simulink model "ardupilotsailboat"  (R2022b)
settings: Solver=VariableStepAuto  StartTime=0.0  StopTime=85  RelTol=1e-3
values from neighbouring files (symbols this model uses):
  m11 = 0.1    [ThreeDOF.m]
  m22 = 0.1    [ThreeDOF.m]
undefined symbols (not defined in the file or in its folder): Ixx, m, Waypoints, Yv
libraries: cstblocks x2, simulink x1
(part 1 of 2)
settings Model: Creator=ruben  LastModifiedBy=ruben
settings SolverCC: MaxConsecutiveZCs=10  MaxConsecutiveMinStep=10  ZeroCrossControl=DisableAll  ZeroCrossAlgorithm=Adaptive  SolverResetMethod=Robust
settings DebuggingCC: SignalInfNanChecking=warning  AlgebraicLoopMsg=error  ArtificialAlgebraicLoopMsg=error  BlockPriorityViolationMsg=error  MinStepSizeMsg=error  MaskedZcDiagnostic=error  IgnoredZcDiagnostic=none  MultiTaskCondExecSysMsg=warning  MultiTaskRateTransMsg=warning  CheckMatrixSingularityMsg=error  StateNameClashWarn=warning

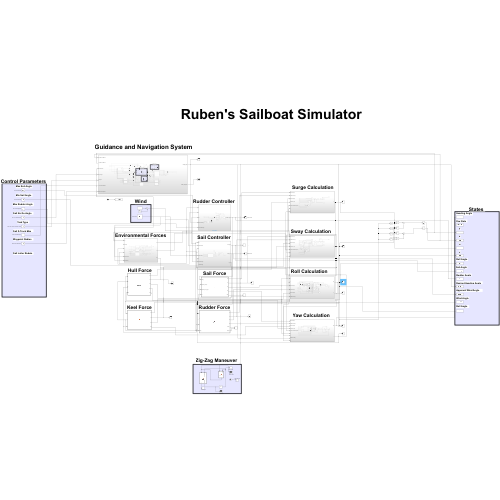
[thumbnail: Simulink's stored preview of the top-level diagram]
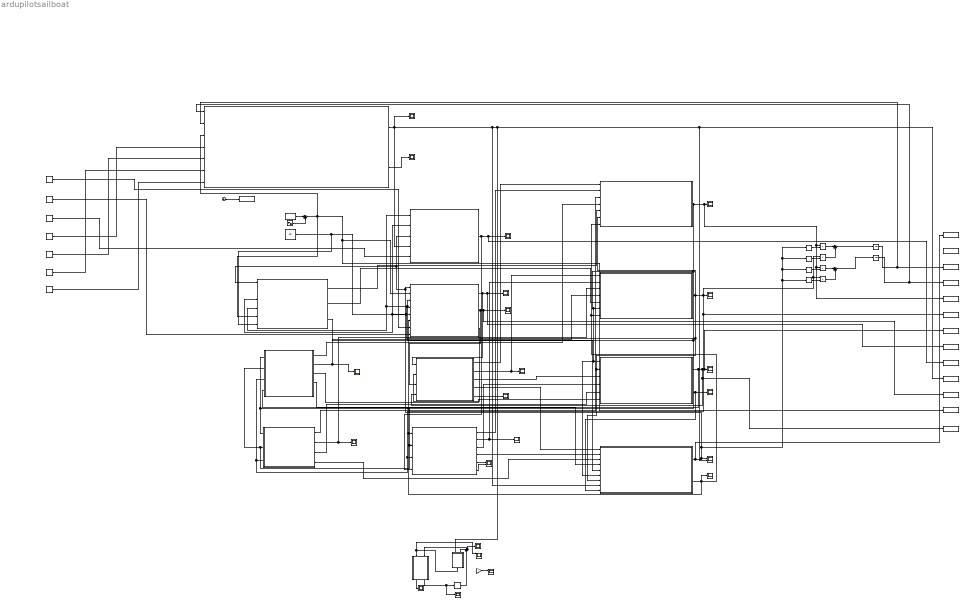
== system ardupilotsailboat ==
  note: Sail Force
  note: Ruben's Sailboat Simulator
  note: States
  note: x
  note: y
  note: Yaw Rate
  note: Heading Angle
  note: u
  note: v
  note: Roll Angle
  note: Sail Angle
  note: Rudder Angle
  note: Desired Heading Angle
  note: Apparent Wind Angle
  note: Wind Angle
  note: Roll Angle
  note: Guidance and Navigation System
  note: Environmental Forces
  note: Surge Calculation
  note: Sway Calculation
  note: Roll Calculation
  note: Yaw Calculation
  note: Wind
  note: Rudder Force
  note: Keel Force
  note: Hull Force
  note: Sail Controller
  note: Rudder Controller
  note: Zig-Zag Maneuver
  note: Control Parameters
  note: Max Sail Angle
  note: Min Sail Angle
  note: Sail No Go Angle
  note: Sail X-Track Max
  note: Sail Loiter Raduis
  note: Waypoint Radius
  note: Tack Type
  note: Max Rudder Angle
  Clock2 : Clock
  Cross-Track Distance(m) : Constant  Value=10
  Delay1 : Delay  DelayLength=1  SampleTime=0.01
  Gain2 : Gain  Gain=180/pi
  Integrator1 : Integrator
  Integrator2 : Integrator
  MATLAB Function3 : MATLAB Function  TreatAsAtomicUnit=on
  MATLAB Function4 : MATLAB Function  TreatAsAtomicUnit=on
  MATLAB Function5 : MATLAB Function  TreatAsAtomicUnit=on
  MATLAB Function6 : MATLAB Function  TreatAsAtomicUnit=on
  MATLAB Function7 : MATLAB Function  TreatAsAtomicUnit=on
  MATLAB Function8 : MATLAB Function  TreatAsAtomicUnit=on
  Product{,1,8..9} (4 alike) : Product
  Radius of Acceptance(m) : Constant  Value=5
  Scope{,1..4,33,35..38,40,42} (12 alike) : Scope
  Scope39 : Scope  NumInputPorts=2
  Scope41 : Scope  NumInputPorts=2
  Sine Wave : Sin  Amplitude=0  Frequency=0.1  SampleTime=0
  Subsystem1 : Subsystem
  Subsystem2 : Subsystem
  Subsystem3 : Subsystem
  Subsystem4 : Subsystem
  Subsystem5 : Subsystem
  Subsystem6 : Subsystem
  Subsystem7 : Subsystem
  Subsystem8 : Subsystem
  Sum : Sum  Inputs=|++
  Sum6 : Sum  Inputs=|+-
  Sum7 : Sum  Inputs=|++
  "Tack Type (1:Direct, 2:Indirect 3:Zone)" : Constant  Value=2
  To Workspace : ToWorkspace  VariableName=yawrate  SaveFormat=Timeseries  SampleTime=-1
  To Workspace1 : ToWorkspace  VariableName=yaw  SaveFormat=Timeseries  SampleTime=-1
  To Workspace10 : ToWorkspace  VariableName=psid  SaveFormat=Timeseries  SampleTime=-1
  To Workspace11 : ToWorkspace  VariableName=awa  SaveFormat=Timeseries  SampleTime=-1
  To Workspace12 : ToWorkspace  VariableName=wind  SaveFormat=Timeseries  SampleTime=-1
  To Workspace13 : ToWorkspace  VariableName=roll  SaveFormat=Timeseries  SampleTime=-1
  To Workspace14 : ToWorkspace  VariableName=time1  SaveFormat=Timeseries  SampleTime=-1
  To Workspace3 : ToWorkspace  VariableName=x  SaveFormat=Timeseries  SampleTime=-1
  To Workspace4 : ToWorkspace  VariableName=y  SaveFormat=Timeseries  SampleTime=-1
  To Workspace5 : ToWorkspace  VariableName=u  SaveFormat=Timeseries  SampleTime=-1
  To Workspace6 : ToWorkspace  VariableName=v  SaveFormat=Timeseries  SampleTime=-1
  To Workspace7 : ToWorkspace  VariableName=phi  SaveFormat=Timeseries  SampleTime=-1
  To Workspace8 : ToWorkspace  VariableName=delta_s  SaveFormat=Timeseries  SampleTime=-1
  To Workspace9 : ToWorkspace  VariableName=delta_r  SaveFormat=Timeseries  SampleTime=-1
  Trigonometric Function : Trigonometry
  Trigonometric Function1 : Trigonometry  Operator=cos
  Trigonometric Function6 : Trigonometry  Operator=cos
  Trigonometric Function7 : Trigonometry
  apparent wind : Scope
  max rudder angle(Rad) : Constant  Value=pi/6
  max sail angle(Rad) : Constant  Value=pi/3
  min sail angle(Rad) : Constant  Value=-pi/3
  rudder and psi1 : Scope  NumInputPorts=2
  rudder angle5 : Scope
  rudder angle6 : Scope
  rudder angle7 : Scope  NumInputPorts=3
  rudder angle8 : Scope
  rudder_angle1 : Scope
  sail angle : Scope
  sail no go angle(Degrees) : Constant  Value=45
  wind direction : Constant  Value=pi/2-0.01
  wind velocity : Constant  Value=10
  wires:
  Trigonometric Function1/1 -> Product/2
  Trigonometric Function/1 -> Product1/2
  Product/1 -> Sum6/1
  Product1/1 -> Sum6/2
  Sum6/1 -> Integrator1/1
  Product9/1 -> Sum7/2
  Product8/1 -> Sum7/1
  Trigonometric Function7/1 -> Product8/2
  Trigonometric Function6/1 -> Product9/2
  Sum7/1 -> Integrator2/1
  Integrator2/1 -> Subsystem1/1(x position of Sailboat), To Workspace3/1
  Integrator1/1 -> Subsystem1/2(y position of Sailboat), To Workspace4/1
  Subsystem1/1(heading (rad)) -> To Workspace10/1, Scope39/2, MATLAB Function8/1(psi), Subsystem6/8(desired heading), Scope/1, Subsystem8/4(desired heading)
  Subsystem1/2(heading (degrees)) -> Scope33/1
  MATLAB Function3/1(Xs) -> Subsystem2/1(sail force (Xs))
  MATLAB Function3/2(Ys) -> Scope1/1, Subsystem4/1(sail force (Ys))
  MATLAB Function3/3(Ks) -> Subsystem5/3(sail force (Ks))
  MATLAB Function3/4(Ns) -> Subsystem6/1(sail force (Ns))
  MATLAB Function4/1(Xr) -> Subsystem2/2(rudder force (Xr))
  MATLAB Function4/2(Yr) -> Scope2/1, Subsystem4/2(rudder force (Yr))
  MATLAB Function4/3(Kr) -> Subsystem5/4(hull force(Kh))
  MATLAB Function4/4(Nr) -> Subsystem6/2(rudder force (Nr))
  MATLAB Function5/1(Xk) -> Subsystem2/3(keel force (Xk))
  MATLAB Function5/2(Yk) -> Scope3/1, Subsystem4/3(keel force (Yk))
  MATLAB Function5/3(Kk) -> Subsystem5/5(keel force (Kk))
  MATLAB Function5/4(Nk) -> Subsystem6/3(keel force (Nk))
  MATLAB Function6/1(Xh) -> Subsystem2/4(hull force (Xh))
  MATLAB Function6/3(Kh) -> Subsystem5/6(rudder force (Kr))
  MATLAB Function6/4(Nh) -> Subsystem6/4(hull force (Nh))
  Subsystem4/1(v) -> To Workspace6/1, MATLAB Function6/3(v), MATLAB Function5/3(v), MATLAB Function4/3(v), Product1/1, Product9/1, Scope36/1, Subsystem2/6(v), Subsystem6/7(v), Subsystem5/2(v), Subsystem8/2(v), Subsystem3/3(v), Subsystem7/4(v)
  Subsystem3/1(Xe) -> Subsystem2/5(environmental force (Xe))
  Subsystem3/2(Ye) -> Subsystem4/5(environmental force (Ye))
  Subsystem3/3(Ne) -> Subsystem6/5(environmental force (Ne))
  Subsystem2/1(u) -> MATLAB Function5/2(u), MATLAB Function6/2(u), MATLAB Function4/2(u), Subsystem8/1(u), Subsystem3/4(u), Subsystem7/3(u), Subsystem6/6(u), Subsystem5/1(u), Subsystem4/6(u), To Workspace5/1, Product8/1, Product/1, Scope35/1
  Subsystem6/2(r) -> Subsystem7/6(r), MATLAB Function5/1(r), MATLAB Function6/1(r), MATLAB Function4/1(r), Scope40/1, Subsystem2/7(r), Subsystem4/7(r)
  Subsystem5/2(p) -> Subsystem6/9(p), Scope38/1
  Subsystem5/1(phi) -> MATLAB Function6/4(phi), To Workspace13/1, MATLAB Function3/4(phi), To Workspace7/1, Scope37/1
  Clock2/1 -> To Workspace14/1
  MATLAB Function7/2(nextState) -> rudder angle5/1, Delay1/1
  Delay1/1 -> rudder angle8/1, MATLAB Function8/2(state), MATLAB Function7/2(currentState)
  MATLAB Function7/1(y) -> rudder angle6/1
  MATLAB Function8/1(y) -> MATLAB Function7/1(r), rudder angle7/1
  Gain2/1 -> rudder and psi1/1
  Sum/1 -> Subsystem3/5(wind Direction), Subsystem1/3(wind Direction), To Workspace12/1, Subsystem7/2(wind direction)
  wind velocity/1 -> Subsystem3/6(wind Velocity), Subsystem7/5(wind velocity)
  Subsystem7/1(sail angle) -> MATLAB Function3/1(delta_s), To Workspace8/1, sail angle/1
  Subsystem7/2(alpha_aw) -> To Workspace11/1, apparent wind/1, MATLAB Function3/3(apparent_wind_angle)
  Subsystem7/3(V_aw) -> MATLAB Function3/2(apparent_velocity)
  Subsystem8/1(rudder angle) -> To Workspace9/1, rudder_angle1/1, MATLAB Function4/4("delta_r ")
  MATLAB Function4/5(delta_r) -> Scope41/1
  MATLAB Function4/6(alpha_a) -> Scope41/2
  MATLAB Function3/5(awa) -> Scope42/1
  Subsystem6/1(psi) -> To Workspace1/1, Trigonometric Function7/1, Trigonometric Function/1, Trigonometric Function1/1, Trigonometric Function6/1, Subsystem7/1(psi), Subsystem3/1(psi), Subsystem8/3(psi), Scope39/1
  MATLAB Function6/2(Yh) -> Subsystem4/4(hull force (Yh)), Scope4/1
  max sail angle(Rad)/1 -> Subsystem7/7(max sail angle)
  min sail angle(Rad)/1 -> Subsystem7/8(min sail angle)
  max rudder angle(Rad)/1 -> Subsystem8/5(max rudder angle)
  sail no go angle(Degrees)/1 -> Subsystem1/4(no go Angle)
  "Tack Type (1:Direct, 2:Indirect 3:Zone)"/1 -> Subsystem1/5(tack Type)
  Cross-Track Distance(m)/1 -> Subsystem1/6(Cross-Track Distance)
  Radius of Acceptance(m)/1 -> Subsystem1/7(radius of acceptance)
  wind direction/1 -> Sum/1
  Sine Wave/1 -> Sum/2

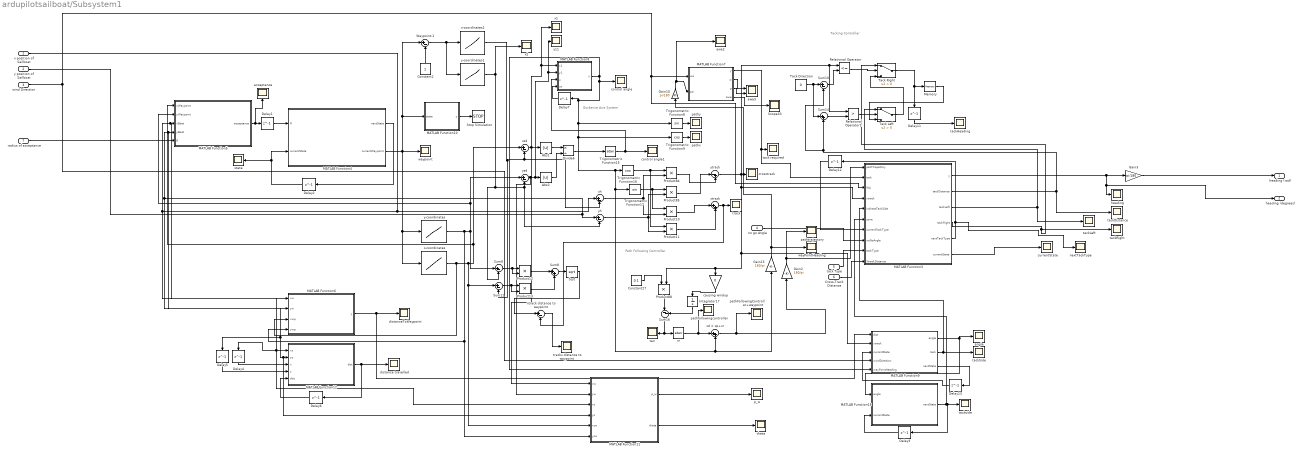
== system ardupilotsailboat/Subsystem1 ==
  note: Guidance Axis System
  note: Tacking Controller
  note: Path Following Controller
  x position of Sailboat : Inport
  y position of Sailboat : Inport  Port=2
  wind Direction : Inport  Port=3
  no go Angle : Inport  Port=4
  tack Type : Inport  Port=5
  Cross-Track Distance : Inport  Port=6
  radius of acceptance : Inport  Port=7
  Abs1 : Abs  SaturateOnIntegerOverflow=off
  Abs2 : Abs  SaturateOnIntegerOverflow=off
  Constant2 : Constant
  Constant27 : Constant  Value=0.1
  Delay{1..2,4..7,11..12} (8 alike) : Delay  DelayLength=1
  Delay13 : Delay  DelayLength=1  SampleTime=2
  Delay3 : Delay  DelayLength=1  SampleTime=2
  Divide6 : Product  Inputs=*/
  Gain10 : Gain  Gain=pi/180
  Gain15 : Gain  Gain=180/pi
  Gain2 : Gain  Gain=180/pi
  Gain3 : Gain  Gain=pi/180
  Integrator17 : Integrator  LimitOutput=on  UpperSaturationLimit=10  LowerSaturationLimit=-10
  MATLAB Function10 : MATLAB Function  TreatAsAtomicUnit=on
  MATLAB Function11 : MATLAB Function  TreatAsAtomicUnit=on
  MATLAB Function12 : MATLAB Function  TreatAsAtomicUnit=on
  MATLAB Function18 : MATLAB Function  TreatAsAtomicUnit=on
  MATLAB Function3 : MATLAB Function  TreatAsAtomicUnit=on
  MATLAB Function4 : MATLAB Function  TreatAsAtomicUnit=on
  MATLAB Function5 : MATLAB Function  TreatAsAtomicUnit=on
  MATLAB Function6 : MATLAB Function  TreatAsAtomicUnit=on
  MATLAB Function7 : MATLAB Function  TreatAsAtomicUnit=on
  MATLAB Function8 : MATLAB Function  TreatAsAtomicUnit=on
  MATLAB Function9 : MATLAB Function  TreatAsAtomicUnit=on
  Memory : Memory
  Product{10..13,84..85,88} (7 alike) : Product
  Relational Operator : RelationalOperator  Operator=<=  OutDataTypeStr=boolean  RndMeth=Simplest  InputSameDT=off
  Relational Operator1 : RelationalOperator  Operator=>  OutDataTypeStr=boolean  RndMeth=Simplest  InputSameDT=off
  Scope33 : Scope
  Sqrt : Sqrt
  Stop Simulation : Stop
  Sum10 : Sum  Inputs=|+-
  Sum11 : Sum  Inputs=|+-
  Sum14 : Sum  Inputs=|++
  Sum16 : Sum  Inputs=|--
  Sum8 : Sum  Inputs=|++
  Sum9 : Sum  Inputs=|+-
  Tack Direction : Constant  Value=0
  Tack Left : Switch  Criteria=u2 > Threshold  SaturateOnIntegerOverflow=off  InputSameDT=off
  Tack Right : Switch  Criteria=u2 > Threshold  SaturateOnIntegerOverflow=off  InputSameDT=off
  Trigonometric Function15 : Trigonometry  Operator=atan
  Trigonometric Function16 : Trigonometry  Operator=cos
  Trigonometric Function17 : Trigonometry
  Trigonometric Function8 : Trigonometry
  Trigonometric Function9 : Trigonometry  Operator=cos
  Waypoint-1 : Sum  Inputs=|+-
  acceptance : Scope
  angle : Scope
  awa2 : Scope
  awa3 : Scope  NumInputPorts=2
  causing windup : Gain  Gain=0
  control angle : Scope
  control angle1 : Scope
  crosstrack : Scope
  currentState : Scope
  distance travelled : Scope
  distanceToWaypoint : Scope
  heading : Scope
  nextTackType : Scope
  p_w : Scope
  "pathFollowingController+waypoint " : Scope
  pathfollowingcontroller : Scope
  pathtrajectory : Scope
  pathx : Scope
  pathy : Scope
  state : Scope
  tack required : Scope
  tackDistance : Scope
  tackHeading : Scope
  tackLeft : Scope
  tackRight : Scope
  tackSide : Scope
  tackside : Scope
  tan : Scope
  theta : Scope
  track : Scope
  trackx distance to waypoint : Scope
  wayPointHeading : Scope
  waypoint : Scope
  x-coordinates : Lookup_n-D  NumberOfTableDimensions=1  BreakpointsForDimension1=Waypoints.number  Table=Waypoints.x  InterpMethod=Cubic spline  ExtrapMethod=Cubic spline  InternalRulePriority=Speed  RndMeth=Simplest
  x-coordinates1 : Lookup_n-D  NumberOfTableDimensions=1  BreakpointsForDimension1=Waypoints.number  Table=Waypoints.x  InterpMethod=Cubic spline  ExtrapMethod=Cubic spline  InternalRulePriority=Speed  RndMeth=Simplest
  x1 : Scope
  x2 : Scope
  xd = xp+xr : Sum  Inputs=|++
  xh : Sum  Inputs=|+-
  xr : Trigonometry  Operator=atan
  xsd : Sum  Inputs=|+-
  xtrack : Sum  Inputs=|++
  xtrack distance to waypoint : Sum  Inputs=|+-
  y-coordinates : Lookup_n-D  NumberOfTableDimensions=1  BreakpointsForDimension1=Waypoints.number  Table=Waypoints.y  InterpMethod=Cubic spline  ExtrapMethod=Cubic spline  InternalRulePriority=Speed  RndMeth=Simplest
  y-coordinates1 : Lookup_n-D  NumberOfTableDimensions=1  BreakpointsForDimension1=Waypoints.number  Table=Waypoints.y  InterpMethod=Cubic spline  ExtrapMethod=Cubic spline  InternalRulePriority=Speed  RndMeth=Simplest
  y11 : Scope
  yh : Sum  Inputs=|+-
  ysd : Sum  Inputs=|+-
  ytrack : Sum  Inputs=|-+
  heading (rad) : Outport
  heading (degrees) : Outport  Port=2
  wires:
  MATLAB Function11/2(theta) -> theta/1
  MATLAB Function7/3(p) -> awa3/2
  Delay2/1 -> MATLAB Function4/2(currentState), state/1
  y-coordinates/1 -> MATLAB Function11/6(ycw), MATLAB Function6/4(ywp), MATLAB Function5/2(yWaypoint), ysd/1, Sum9/1
  Trigonometric Function17/1 -> Product10/1, Product85/1
  MATLAB Function3/6(currentState) -> currentState/1
  MATLAB Function3/1(y) -> heading (degrees)/1, heading/1, Gain3/1
  Gain2/1 -> MATLAB Function3/1(pathTrajectory), pathtrajectory/1
  Delay12/1 -> MATLAB Function3/7(currentTackType)
  MATLAB Function4/2(currentWaypoint) -> MATLAB Function10/1(state), Waypoint-1/1, waypoint/1, x-coordinates/1, y-coordinates/1
  yh/1 -> Product85/2, Product11/2
  MATLAB Function7/2(w) -> awa3/1
  Sum14/1 -> Relational Operator1/2
  y position of Sailboat/1 -> yh/1, MATLAB Function6/2(yw), MATLAB Function5/4(yBoat), MATLAB Function11/4(ys), MATLAB Function12/2(ys), Delay5/1
  ytrack/1 -> MATLAB Function3/4(xtrack), Product88/2, causing windup/1, MATLAB Function9/2(xtrack), crosstrack/1, Relational Operator1/1, Relational Operator/1
  Product85/1 -> ytrack/1
  Delay11/1 -> tackHeading/1
  MATLAB Function3/2(tackDistance) -> Sum10/2, Sum14/2, tackDistance/1
  Integrator17/1 -> Sum16/2
  Abs1/1 -> Divide6/1
  Trigonometric Function16/1 -> Product11/1, Product84/1
  Delay7/1 -> MATLAB Function8/4(us)
  MATLAB Function18/1(nextState) -> tackside/1, Delay3/1, MATLAB Function3/6(zone)
  xd = xp+xr/1 -> "pathFollowingController+waypoint "/1, Gain2/1
  Gain10/1 -> MATLAB Function7/2(psi), awa2/1
  MATLAB Function3/5(nextTackType) -> nextTackType/1, Delay12/1
  Delay13/1 -> MATLAB Function9/3(currentState)
  Waypoint-1/1 -> x-coordinates1/1, y-coordinates1/1
  Delay3/1 -> MATLAB Function18/2(currentState)
  xsd/1 -> MATLAB Function11/1(xw), MATLAB Function8/1(x1), x1/1, Abs1/1
  Constant2/1 -> Waypoint-1/2
  MATLAB Function8/1(y) -> Trigonometric Function8/1, Trigonometric Function9/1, Trigonometric Function17/1, xd = xp+xr/2, Gain15/1, Trigonometric Function16/1, Delay7/1, control angle/1, MATLAB Function9/5(wayPointHeading)
  xh/1 -> Product84/2, Product10/2
  Delay1/1 -> MATLAB Function4/1(R)
  MATLAB Function9/3(nextState) -> Delay13/1
  Product84/1 -> ytrack/2
  y-coordinates1/1 -> yh/2, ysd/2, Sum9/2, x2/1
  x position of Sailboat/1 -> xh/1, MATLAB Function11/3(xs), MATLAB Function12/1(xs), Delay4/1, MATLAB Function6/1(xw), MATLAB Function5/3(xBoat)
  Trigonometric Function15/1 -> control angle1/1, MATLAB Function8/3(u)
  ysd/1 -> y11/1, MATLAB Function8/2(y1), Abs2/1, MATLAB Function11/2(yw)
  x-coordinates1/1 -> Sum11/2, xh/2, xsd/2
  Sum16/1 -> xr/1, tan/1
  Divide6/1 -> Trigonometric Function15/1
  Product13/1 -> Sum8/2
  Gain15/1 -> Gain10/1, wayPointHeading/1
  MATLAB Function6/1(y) -> MATLAB Function9/1(dist), distanceToWaypoint/1
  Delay5/1 -> MATLAB Function12/4(y)
  MATLAB Function9/1(angle) -> angle/1, MATLAB Function18/1(angle)
  Product88/1 -> Sum16/1
  Relational Operator1/1 -> Tack Left/2
  MATLAB Function3/3(tackLeft) -> Tack Left/1, tackLeft/1
  Tack Right/1 -> Memory/1, Delay11/1
  xtrack distance to waypoint/1 -> trackx distance to waypoint/1
  x-coordinates/1 -> MATLAB Function6/3(xwp), MATLAB Function11/5(xcw), Sum11/1, xsd/1, MATLAB Function5/1(xWaypoint)
  Constant27/1 -> Product88/1
  Memory/1 -> Tack Left/3
  Product11/1 -> xtrack/2
  Trigonometric Function8/1 -> pathy/1
  MATLAB Function7/1(y) -> MATLAB Function3/2(tack), tack required/1
  Delay4/1 -> MATLAB Function12/3(x)
  causing windup/1 -> Integrator17/1
  Tack Left/1 -> Tack Right/3
  MATLAB Function9/2(tack) -> MATLAB Function3/5(indirectTackSide), tackSide/1
  MATLAB Function10/1(y) -> Stop Simulation/1
  wind Direction/1 -> MATLAB Function3/3(WA), MATLAB Function7/1(wa), MATLAB Function9/4(windDirection)
  Sum8/1 -> Sqrt/1
  Sum11/1 -> Product13/2, Product13/1
  Tack Direction/1 -> Sum14/1, Sum10/1
  Sum9/1 -> Product12/1, Product12/2
  Delay6/1 -> MATLAB Function12/5("dist ")
  MATLAB Function5/1(acceptance) -> acceptance/1, Delay1/1
  MATLAB Function12/1(dist) -> distance travelled/1, Delay6/1
  Relational Operator/1 -> Tack Right/2
  Sum10/1 -> Relational Operator/2
  xtrack/1 -> xtrack distance to waypoint/2, track/1
  Abs2/1 -> Divide6/2
  MATLAB Function4/1(nextState) -> Delay2/1
  Sqrt/1 -> xtrack distance to waypoint/1
  MATLAB Function11/1(p_w) -> p_w/1
  Product10/1 -> xtrack/1
  xr/1 -> xd = xp+xr/1, pathfollowingcontroller/1
  MATLAB Function3/4(tackRight) -> Tack Right/1, tackRight/1
  Product12/1 -> Sum8/1
  Trigonometric Function9/1 -> pathx/1
  Gain3/1 -> heading (rad)/1
  MATLAB Function7/4(awa) -> Scope33/1
  no go Angle/1 -> MATLAB Function3/8(noGoAngle)
  tack Type/1 -> MATLAB Function3/9(tackType)
  Cross-Track Distance/1 -> MATLAB Function3/10(XtrackDistance)
  radius of acceptance/1 -> MATLAB Function5/5(R)

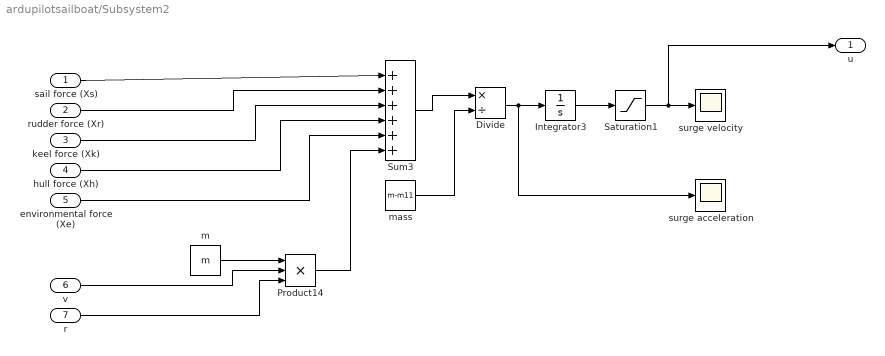
== system ardupilotsailboat/Subsystem2 ==
  sail force (Xs) : Inport
  rudder force (Xr) : Inport  Port=2
  keel force (Xk) : Inport  Port=3
  hull force (Xh) : Inport  Port=4
  environmental force (Xe) : Inport  Port=5
  v : Inport  Port=6
  r : Inport  Port=7
  Divide : Product  Inputs=*/
  Integrator3 : Integrator  InitialCondition=1.3
  Product14 : Product  Inputs=3
  Saturation1 : Saturate  UpperLimit=1.3  LowerLimit=-1.3
  Sum3 : Sum  Inputs=|++++++
  m : Constant  Value=m
  mass : Constant  Value=m-m11
  surge acceleration : Scope
  surge velocity : Scope
  u : Outport
  wires:
  Saturation1/1 -> u/1, surge velocity/1
  sail force (Xs)/1 -> Sum3/1
  Integrator3/1 -> Saturation1/1
  m/1 -> Product14/1
  Divide/1 -> surge acceleration/1, Integrator3/1
  mass/1 -> Divide/2
  Sum3/1 -> Divide/1
  Product14/1 -> Sum3/6
  rudder force (Xr)/1 -> Sum3/2
  keel force (Xk)/1 -> Sum3/3
  hull force (Xh)/1 -> Sum3/4
  environmental force (Xe)/1 -> Sum3/5
  v/1 -> Product14/2
  r/1 -> Product14/3

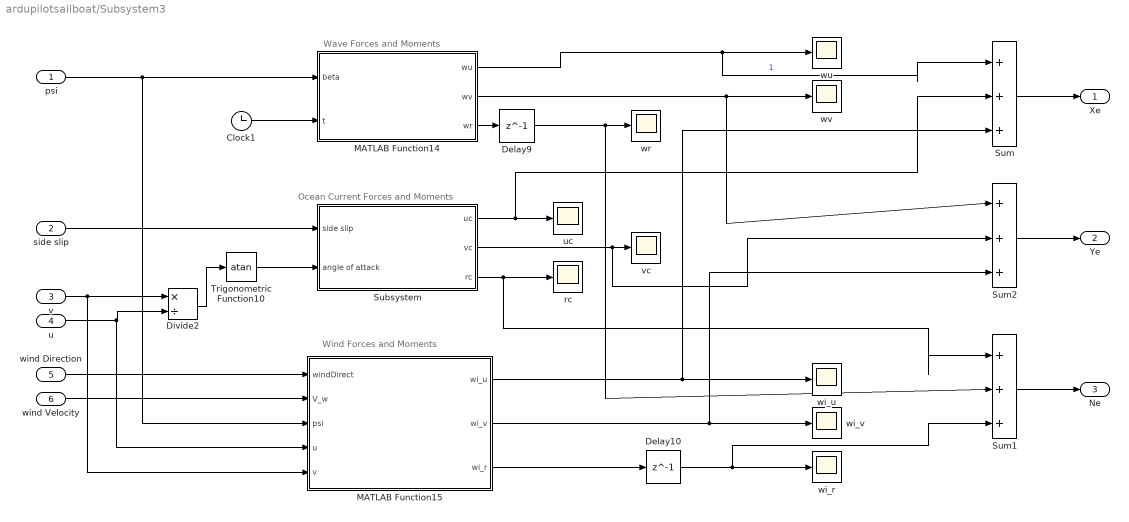
== system ardupilotsailboat/Subsystem3 ==
  note: Wave Forces and Moments
  note: Wind Forces and Moments
  note: Ocean Current Forces and Moments
  psi : Inport
  side slip : Inport  Port=2
  v : Inport  Port=3
  u : Inport  Port=4
  wind Direction : Inport  Port=5
  wind Velocity : Inport  Port=6
  Clock1 : Clock
  Delay10 : Delay  DelayLength=1
  Delay9 : Delay  DelayLength=1
  Divide2 : Product  Inputs=*/
  MATLAB Function14 : MATLAB Function  TreatAsAtomicUnit=on
  MATLAB Function15 : MATLAB Function  TreatAsAtomicUnit=on
  Subsystem : Subsystem
  Sum : Sum  Inputs=|+++
  Sum1 : Sum  Inputs=|+++
  Sum2 : Sum  Inputs=|+++
  Trigonometric Function10 : Trigonometry  Operator=atan
  rc : Scope
  uc : Scope
  vc : Scope
  wi_r : Scope
  wi_u : Scope
  wi_v : Scope
  wr : Scope
  wu : Scope
  wv : Scope
  Xe : Outport
  Ye : Outport  Port=2
  Ne : Outport  Port=3
  wires:
  MATLAB Function14/2(wv) -> Sum2/1, wv/1
  Trigonometric Function10/1 -> Subsystem/2(angle of attack)
  MATLAB Function14/3(wr) -> Delay9/1
  MATLAB Function15/2(wi_v) -> Sum2/3, wi_v/1
  Subsystem/1(uc) -> Sum/2, uc/1
  MATLAB Function15/3(wi_r) -> Delay10/1
  MATLAB Function15/1(wi_u) -> Sum/3, wi_u/1
  Clock1/1 -> MATLAB Function14/2(t)
  Subsystem/2(vc) -> Sum2/2, vc/1
  MATLAB Function14/1(wu) -> Sum/1, wu/1  "1"
  Divide2/1 -> Trigonometric Function10/1
  psi/1 -> MATLAB Function14/1(beta), MATLAB Function15/3(psi)
  side slip/1 -> Subsystem/1(side slip)
  v/1 -> MATLAB Function15/5(v), Divide2/1
  u/1 -> MATLAB Function15/4(u), Divide2/2
  wind Direction/1 -> MATLAB Function15/1(windDirect)
  wind Velocity/1 -> MATLAB Function15/2(V_w)
  Sum/1 -> Xe/1
  Sum1/1 -> Ne/1
  Sum2/1 -> Ye/1
  Delay10/1 -> Sum1/3, wi_r/1
  Subsystem/3(rc) -> Sum1/1, rc/1
  Delay9/1 -> Sum1/2, wr/1

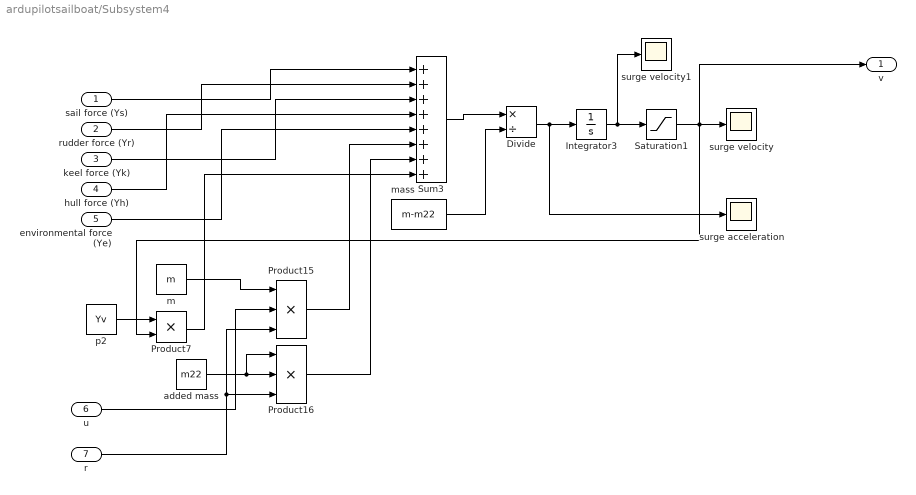
== system ardupilotsailboat/Subsystem4 ==
  sail force (Ys) : Inport
  rudder force (Yr) : Inport  Port=2
  keel force (Yk) : Inport  Port=3
  hull force (Yh) : Inport  Port=4
  environmental force (Ye) : Inport  Port=5
  u : Inport  Port=6
  r : Inport  Port=7
  Divide : Product  Inputs=*/
  Integrator3 : Integrator  LimitOutput=on  UpperSaturationLimit=0.05  LowerSaturationLimit=-0.05
  Product15 : Product  Inputs=3
  Product16 : Product  Inputs=3
  Product7 : Product
  Saturation1 : Saturate  UpperLimit=0.1  LowerLimit=-0.1
  Sum3 : Sum  Inputs=|++++++++
  added mass : Constant  Value=m22
  m : Constant  Value=m
  mass : Constant  Value=m-m22
  p2 : Constant  Value=Yv
  surge acceleration : Scope
  surge velocity : Scope
  surge velocity1 : Scope
  v : Outport
  wires:
  Saturation1/1 -> Product7/2, v/1, surge velocity/1
  sail force (Ys)/1 -> Sum3/1
  Integrator3/1 -> surge velocity1/1, Saturation1/1
  Divide/1 -> surge acceleration/1, Integrator3/1
  mass/1 -> Divide/2
  Sum3/1 -> Divide/1
  rudder force (Yr)/1 -> Sum3/2
  keel force (Yk)/1 -> Sum3/3
  hull force (Yh)/1 -> Sum3/4
  environmental force (Ye)/1 -> Sum3/5
  added mass/1 -> Product16/1, Product16/2
  p2/1 -> Product7/1
  m/1 -> Product15/1
  Product15/1 -> Sum3/6
  Product16/1 -> Sum3/7
  u/1 -> Product15/2
  Product7/1 -> Sum3/8
  r/1 -> Product16/3, Product15/3

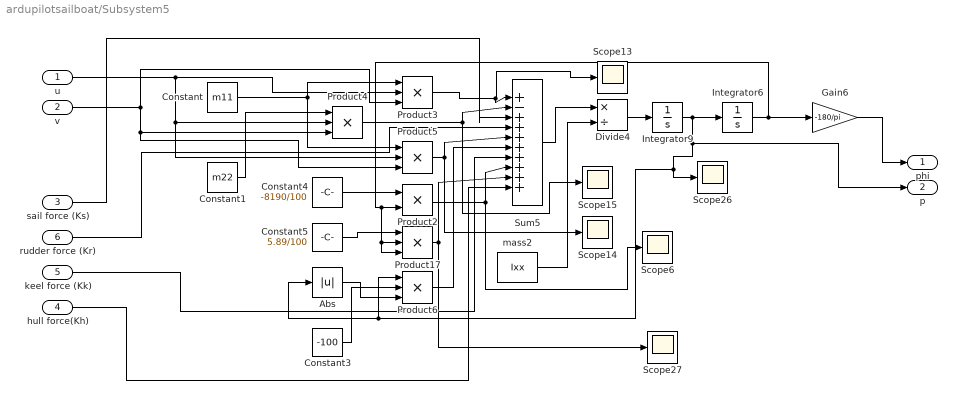
== system ardupilotsailboat/Subsystem5 ==
  u : Inport
  v : Inport  Port=2
  sail force (Ks) : Inport  Port=3
  hull force(Kh) : Inport  Port=4
  keel force (Kk) : Inport  Port=5
  rudder force (Kr) : Inport  Port=6
  Abs : Abs  SaturateOnIntegerOverflow=off
  Constant : Constant  Value=m11
  Constant1 : Constant  Value=m22
  Constant3 : Constant  Value=-100
  Constant4 : Constant  Value=-8190/100
  Constant5 : Constant  Value=5.89/100
  Divide4 : Product  Inputs=*/
  Gain6 : Gain  Gain=-180/pi
  Integrator6 : Integrator
  Integrator9 : Integrator
  Product{3..6,17} (5 alike) : Product  Inputs=3
  Product2 : Product
  Scope{6,13..15,26..27} (6 alike) : Scope
  Sum5 : Sum  Inputs=|+-++++++++
  mass2 : Constant  Value=Ixx
  phi : Outport
  p : Outport  Port=2
  wires:
  Product6/1 -> Sum5/6
  Abs/1 -> Product6/3
  Product4/1 -> Scope15/1, Sum5/2
  Constant3/1 -> Product6/2
  Integrator9/1 -> p/1, Abs/1, Product6/1, Scope26/1, Integrator6/1
  Integrator6/1 -> Product2/2, Product17/3, Product17/2, Gain6/1
  Product17/1 -> Sum5/9, Scope27/1
  Product2/1 -> Scope6/1, Sum5/8
  Constant/1 -> Product5/1, Product3/1
  Product3/1 -> Sum5/1, Scope13/1
  Constant5/1 -> Product17/1
  Product5/1 -> Scope14/1, Sum5/5
  Constant4/1 -> Product2/1
  Divide4/1 -> Integrator9/1
  mass2/1 -> Divide4/2
  Constant1/1 -> Product4/1
  Sum5/1 -> Divide4/1
  u/1 -> Product5/2, Product4/2, Product3/2
  v/1 -> Product3/3, Product5/3, Product4/3
  sail force (Ks)/1 -> Sum5/3
  rudder force (Kr)/1 -> Sum5/4
  keel force (Kk)/1 -> Sum5/7
  hull force(Kh)/1 -> Sum5/10
  Gain6/1 -> phi/1

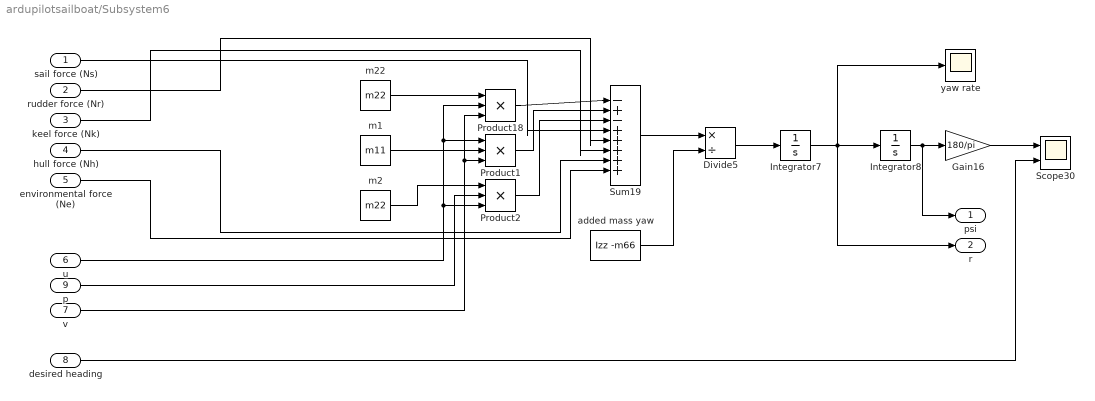
== system ardupilotsailboat/Subsystem6 ==
  sail force (Ns) : Inport
  rudder force (Nr) : Inport  Port=2
  keel force (Nk) : Inport  Port=3
  hull force (Nh) : Inport  Port=4
  environmental force (Ne) : Inport  Port=5
  u : Inport  Port=6
  v : Inport  Port=7
  desired heading : Inport  Port=8
  p : Inport  Port=9
  Divide5 : Product  Inputs=*/
  Gain16 : Gain  Gain=180/pi
  Integrator7 : Integrator
  Integrator8 : Integrator
  Product1 : Product  Inputs=3
  Product18 : Product  Inputs=3
  Product2 : Product  Inputs=3
  Scope30 : Scope  NumInputPorts=2
  Sum19 : Sum  Inputs=|-+-+++++
  added mass yaw : Constant  Value=Izz -m66
  m1 : Constant  Value=m11
  m2 : Constant  Value=m22
  m22 : Constant  Value=m22
  yaw rate : Scope
  psi : Outport
  r : Outport  Port=2
  wires:
  Product18/1 -> Sum19/1
  Gain16/1 -> Scope30/1
  Product2/1 -> Sum19/3
  m22/1 -> Product18/1
  added mass yaw/1 -> Divide5/2
  m1/1 -> Product1/2
  Product1/1 -> Sum19/2
  Sum19/1 -> Divide5/1
  Integrator7/1 -> r/1, yaw rate/1, Integrator8/1
  Divide5/1 -> Integrator7/1
  sail force (Ns)/1 -> Sum19/4
  rudder force (Nr)/1 -> Sum19/5
  keel force (Nk)/1 -> Sum19/6
  hull force (Nh)/1 -> Sum19/7
  environmental force (Ne)/1 -> Sum19/8
  u/1 -> Product18/2, Product1/1, Product2/3
  v/1 -> Product1/3, Product18/3
  m2/1 -> Product2/1
  desired heading/1 -> Scope30/2
  Integrator8/1 -> psi/1, Gain16/1
  p/1 -> Product2/2

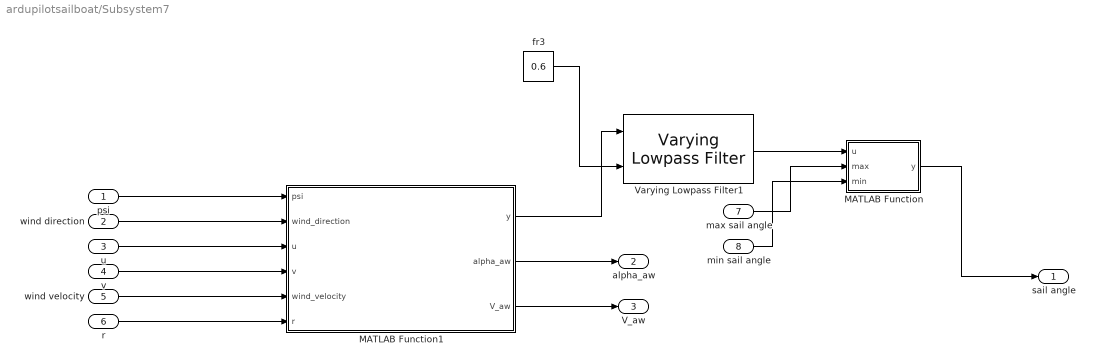
== system ardupilotsailboat/Subsystem7 ==
  psi : Inport
  wind direction : Inport  Port=2
  u : Inport  Port=3
  v : Inport  Port=4
  wind velocity : Inport  Port=5
  r : Inport  Port=6
  max sail angle : Inport  Port=7
  min sail angle : Inport  Port=8
  MATLAB Function : MATLAB Function  TreatAsAtomicUnit=on
  MATLAB Function1 : MATLAB Function  TreatAsAtomicUnit=on
  Varying Lowpass Filter1 : cstblocks/Linear Parameter Varying/Varying Lowpass Filter  N=1
  fr3 : Constant  Value=0.6
  sail angle : Outport
  alpha_aw : Outport  Port=2
  V_aw : Outport  Port=3
  wires:
  MATLAB Function1/1(y) -> Varying Lowpass Filter1/1
  fr3/1 -> Varying Lowpass Filter1/2
  r/1 -> MATLAB Function1/6(r)
  wind velocity/1 -> MATLAB Function1/5(wind_velocity)
  v/1 -> MATLAB Function1/4(v)
  u/1 -> MATLAB Function1/3(u)
  wind direction/1 -> MATLAB Function1/2(wind_direction)
  psi/1 -> MATLAB Function1/1(psi)
  MATLAB Function/1(y) -> sail angle/1
  MATLAB Function1/2(alpha_aw) -> alpha_aw/1
  MATLAB Function1/3(V_aw) -> V_aw/1
  Varying Lowpass Filter1/1 -> MATLAB Function/1(u)
  max sail angle/1 -> MATLAB Function/2(max)
  min sail angle/1 -> MATLAB Function/3(min)

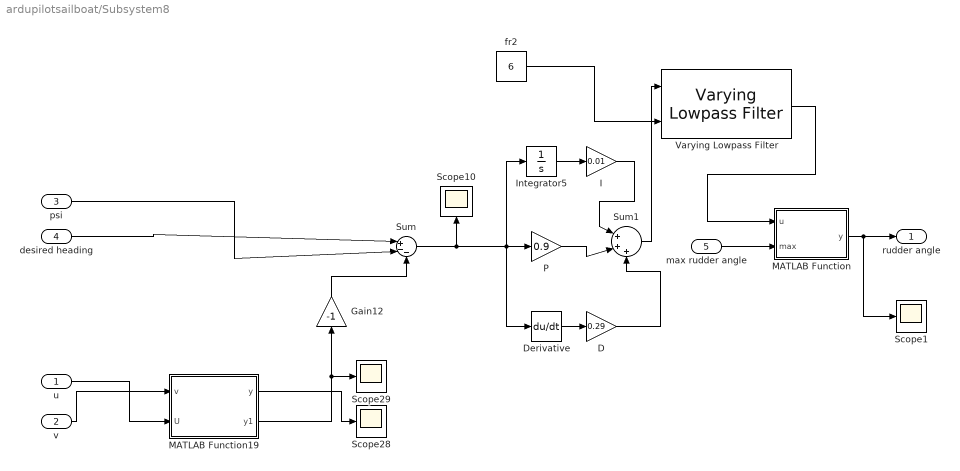
== system ardupilotsailboat/Subsystem8 ==
  u : Inport
  v : Inport  Port=2
  psi : Inport  Port=3
  desired heading : Inport  Port=4
  max rudder angle : Inport  Port=5
  D : Gain  Gain=0.29
  Derivative : Derivative
  Gain12 : Gain  Gain=-1
  I : Gain  Gain=0.01
  Integrator5 : Integrator
  MATLAB Function : MATLAB Function  TreatAsAtomicUnit=on
  MATLAB Function19 : MATLAB Function  TreatAsAtomicUnit=on
  P : Gain  Gain=0.9
  Scope{1,10,28..29} (4 alike) : Scope
  Sum : Sum  Inputs=|+--
  Sum1 : Sum  Inputs=|+++
  Varying Lowpass Filter : cstblocks/Linear Parameter Varying/Varying Lowpass Filter  N=1
  fr2 : Constant  Value=6
  rudder angle : Outport
  wires:
  Varying Lowpass Filter/1 -> MATLAB Function/1(u)
  MATLAB Function/1(y) -> Scope1/1, rudder angle/1
  Sum1/1 -> Varying Lowpass Filter/1
  I/1 -> Sum1/1
  Sum/1 -> Scope10/1, Derivative/1, Integrator5/1, P/1
  fr2/1 -> Varying Lowpass Filter/2
  D/1 -> Sum1/3
  P/1 -> Sum1/2
  Derivative/1 -> D/1
  Integrator5/1 -> I/1
  MATLAB Function19/2(y1) -> Gain12/1, Scope29/1
  MATLAB Function19/1(y) -> Scope28/1
  Gain12/1 -> Sum/3
  u/1 -> MATLAB Function19/2(U)
  v/1 -> MATLAB Function19/1(v)
  psi/1 -> Sum/2
  desired heading/1 -> Sum/1
  max rudder angle/1 -> MATLAB Function/2(max)

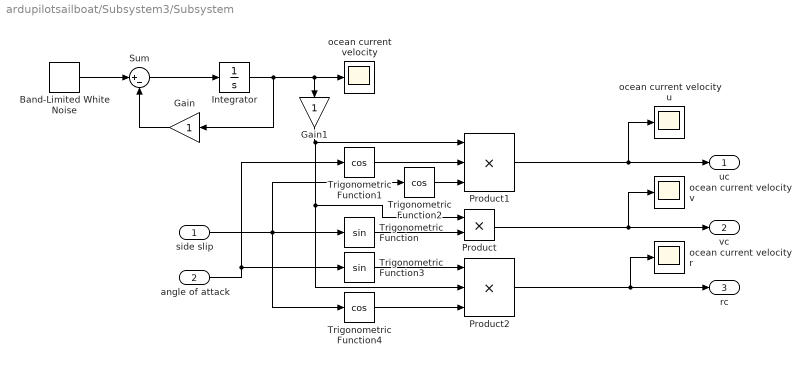
== system ardupilotsailboat/Subsystem3/Subsystem ==
  side slip : Inport
  angle of attack : Inport  Port=2
  Band-Limited White Noise : simulink/Sources/Band-Limited White Noise  Cov=[0.03]  Ts=1  seed=[23341]
  Gain : Gain
  Gain1 : Gain
  Integrator : Integrator
  Product : Product
  Product1 : Product  Inputs=3
  Product2 : Product  Inputs=3
  Sum : Sum  Inputs=|+-
  Trigonometric Function : Trigonometry
  Trigonometric Function1 : Trigonometry  Operator=cos
  Trigonometric Function2 : Trigonometry  Operator=cos
  Trigonometric Function3 : Trigonometry
  Trigonometric Function4 : Trigonometry  Operator=cos
  ocean current velocity : Scope
  ocean current velocity r : Scope
  ocean current velocity u : Scope
  ocean current velocity v : Scope
  uc : Outport
  vc : Outport  Port=2
  rc : Outport  Port=3
  wires:
  Sum/1 -> Integrator/1
  Band-Limited White Noise/1 -> Sum/1
  Integrator/1 -> ocean current velocity/1, Gain1/1, Gain/1
  Gain/1 -> Sum/2
  Trigonometric Function/1 -> Product/2
  side slip/1 -> Trigonometric Function4/1, Trigonometric Function2/1, Trigonometric Function/1
  Product/1 -> ocean current velocity v/1, vc/1
  Trigonometric Function2/1 -> Product1/3
  Trigonometric Function1/1 -> Product1/2
  Product1/1 -> ocean current velocity u/1, uc/1
  Trigonometric Function3/1 -> Product2/1
  Trigonometric Function4/1 -> Product2/3
  angle of attack/1 -> Trigonometric Function3/1, Trigonometric Function1/1
  Product2/1 -> rc/1, ocean current velocity r/1
  Gain1/1 -> Product1/1, Product2/2, Product/1

== matlab function ardupilotsailboat/MATLAB Function4 ==
  data: r input; u input; Xr output; v input; Yr output; Kr output; Nr output; delta_r input; delta_r output; alpha_a output
function [Xr,Yr,Kr,Nr,delta_r,alpha_a] = rudderForce(r,u,v,delta_r)
%Parameters
rudder_width = 4;
rudder_length = 20;
rho_w = 1025;
area = rudder_length * rudder_width * 10^(-4);
velocity = sqrt(v^2+u^2);
l4 = 0.48;
h3 = 0.2;
yr = 0;
xr = -0.5;
zr = 0.2;

% Calculate Angle of Attack
v_aru = -u;
v_arv = -v-r;
alpha_ar = atan2(real(v_arv),real(v_aru));
alpha_a = alpha_ar - delta_r;

% Lift and Drag Coeff
[lc, dc] = ruddercoef(alpha_a);


% Calculate Lift and Drag Force
lift_force = 0.5 * rho_w * area * lc * velocity^2 ;
drag_force = 0.5 * rho_w * area * dc * velocity^2 ;

Xr = (lift_force * sin(alpha_ar) - drag_force * cos(alpha_ar));
Yr = (lift_force * cos(alpha_ar) + drag_force * sin(alpha_ar));
Kr =( h3 * ( -lift_force * cos(alpha_ar) - drag_force * sin(alpha_ar)));
Nr = (l4 * (lift_force * cos(alpha_ar) + drag_force * sin(alpha_ar)));


function [Clr,Cdr] = ruddercoef(attack)
% generate a lookup table for the lift/drag coefficients for the sail
% and compute Cls/Cds from the lookup table using interpolation.

% lookup table
xdata = linspace(-pi,pi,73); % every 5 degrees
xdata = xdata/pi*180;

% lift curve
yl = fliplr([0 0.42 0.73 ...
    0.95 1.1 1.165 1.18 1.155 1.12 1.065 1 0.92 0.83 0.72 0.62 0.48 0.33 0.16])*(-1);
yldata = [fliplr([0 0.42 0.73 ...
    0.95 1.1 1.165 1.18 1.155 1.12 1.065 1 0.92 0.83 0.72 0.62 0.48 0.33 0.16 0 yl])*(-1) ...
    [0.42 0.73 ...
    0.95 1.1 1.165 1.18 1.155 1.12 1.065 1 0.92 0.83 0.72 0.62 0.48 0.33 0.16 0 yl]];

% drag curve
yd = fliplr([0 0.03 0.06 ...
    0.1 0.17 0.3 0.48 0.74 0.98 1.18 1.34 1.5 1.65 1.76 1.89 1.97 2.01 2.05]);
yddata = [fliplr([0 0.03 0.06 ...
    0.1 0.17 0.3 0.48 0.74 0.98 1.18 1.34 1.5 1.65 1.76 1.89 1.97 2.01 2.05 2.08 yd])...
    [0.03 0.06 ...
    0.1 0.17 0.3 0.48 0.74 0.98 1.18 1.34 1.5 1.65 1.76 1.89 1.97 2.01 2.05 2.08 yd]];

% fit the input angle of attack into the interval [-pi,pi]
if attack > pi
    attack = mod(attack+pi,2*pi) - pi;
else
    if attack < -pi
        attack = mod(attack-pi,-2*pi) + pi;
    end
end

% interpolation
attack = attack/pi*180;
Clr = interp1(xdata,yldata,attack,'pchip');
Cdr = interp1(xdata,yddata,attack,'pchip');

== matlab function ardupilotsailboat/MATLAB Function5 ==
  data: r input; u input; Xk output; v input; Yk output; Kk output; Nk output
function [Xk,Yk,Kk,Nk] = keelForce(r,u,v)
%Parameters
keel_width = 8;
keel_length = 45;
rho_w = 1025;
area = keel_width * keel_length * 10^(-4);
velocity = sqrt(v^2+u^2);
l3 = 0.1;
h2 = 0.275;
yk=0;
xk=0.1;
zk=0.25;

% Calculate Angle of Attack
v_aku = -u + r*yk;
v_akv = -v - r*xk + 0*zk;
alpha_ak = atan2(real(v_akv),real(-v_aku));
alpha = alpha_ak;

% Lift and Drag Coeff
[lc, dc] = keelcoef(alpha);

% Calculate Lift and Drag Force
lift_force = 0.5 * rho_w * area * lc * (v_aku^2+v_akv^2);
drag_force = 0.5 * rho_w * area * dc * (v_aku^2+v_akv^2);

Xk = (-lift_force * sin(alpha_ak) + drag_force * cos(alpha_ak));
Yk = (-lift_force * cos(alpha_ak) - drag_force * sin(alpha_ak));
Kk = -(-lift_force*cos(alpha_ak)-drag_force*sin(alpha_ak))*zk;
Nk = -(lift_force*cos(alpha_ak)+drag_force*sin(alpha_ak))*xk;



%------------------------------------------------------------------------------------------------------------------------------
function [Clk,Cdk] = keelcoef(attack)
% generate a lookup table for the lift/drag coefficients for the sail
% and compute Cls/Cds from the lookup table using interpolation.

% lookup table
xdata = linspace(-pi,pi,73); % every 5 degrees
xdata = xdata/pi*180;

% lift curve
yl = fliplr([0 0.425 0.74 ...
    0.94 1.1 1.17 1.19 1.16 1.12 1.07 0.99 0.92 0.84 0.74 0.63 0.49 0.345 0.185])*(-1);
yldata = [fliplr([0 0.425 0.74 ...
    0.94 1.1 1.17 1.19 1.16 1.12 1.07 0.99 0.92 0.84 0.74 0.63 0.49 0.345 0.185 0 yl])*(-1) ...
    [0.425 0.74 ...
    0.94 1.1 1.17 1.19 1.16 1.12 1.07 0.99 0.92 0.84 0.74 0.63 0.49 0.345 0.185 0 yl]];

% drag curve
yd = fliplr([0 0.04 0.07 ...
    0.1 0.17 0.3 0.49 0.76 0.98 1.19 1.34 1.5 1.65 1.77 1.88 1.96 2.01 2.05]);
yddata = [fliplr([0 0.04 0.07 ...
    0.1 0.17 0.3 0.49 0.76 0.98 1.19 1.34 1.5 1.65 1.77 1.88 1.96 2.01 2.05 2.09 yd])...
    [0.04 0.07 ...
    0.1 0.17 0.3 0.49 0.76 0.98 1.19 1.34 1.5 1.65 1.77 1.88 1.96 2.01 2.05 2.09 yd]];

% fit the input angle of attack into the interval [-pi,pi]
if attack > pi
    attack = mod(attack+pi,2*pi) - pi;
else
    if attack < -pi
        attack = mod(attack-pi,-2*pi) + pi;
    end
end

% interpolation
attack = attack/pi*180;
Clk = interp1(xdata,yldata,attack,'pchip');
Cdk = interp1(xdata,yddata,attack,'pchip');


%------------------------------------------------------------------------------------------------------------------------------
function F = resistancehull(alpha_a)

xdata = linspace(0,6,13); % every 0.5m/s
ydata = [0 0.15 0.35 0.5 0.675 0.825 1.175 1.4 2 4.85 9.85 18.46 27.5]*1000;

% interpolation
if alpha_a <= 6
    F = interp1(xdata,ydata,alpha_a,'pchip');
else
    F = interp1(xdata,ydata,alpha_a,'pchip','extrap');
end

== matlab function ardupilotsailboat/MATLAB Function6 ==
  data: r input; u input; Xh output; v input; Yh output; Kh output; Nh output; Frh output; phi input
function [Xh,Yh,Kh,Nh,Frh] = hullForce(r,u,v,phi)
yh=0;
zh=-0.1;
xh=0;
% from the hull
v_ahu = -u + r*yh;
v_ahv = (-v-r*xh + 0*zh)/cos(0);
v_ah = sqrt(v_ahu^2+v_ahv^2);
alpha_ah = atan2(real(v_ahv),real(-v_ahu));
Frh = resistancehull(v_ah);

Xh = Frh*cos(alpha_ah)*2;
Yh = -Frh*sin(alpha_ah)*cos(phi)*100;
Kh = Frh*sin(alpha_ah)*cos(phi)*zh;
Nh = -Frh*sin(alpha_ah)*cos(0)*xh;
%D_hull = [Frh*cos(alpha_ah);-Frh*sin(alpha_ah)*cos(phi); Frh*sin(alpha_ah)*cos(phi)*par.zh; -Frh*sin(alpha_ah)*cos(phi)*par.xh];


function F = resistancehull(alpha_a)

xdata = linspace(0,0.15,13); % every 0.1m/s
ydata = [0 0.075 0.175 0.25 0.3375 0.4125 0.5875 0.7 1 2.425 4.925 9.23 13.75]*0.08;

% interpolation
if alpha_a <= 0.15
    F = interp1(xdata,ydata,alpha_a,'pchip');
else
    F = interp1(xdata,ydata,alpha_a,'pchip','extrap');
end

== matlab function ardupilotsailboat/Subsystem8/MATLAB Function19 ==
  data: y output; v input; U input; y1 output
function [y,y1]     = beta(v,U)
% Beta Reference Angle
y=0;
y1 = real(asin(complex(v/U)));

== matlab function ardupilotsailboat/Subsystem7/MATLAB Function1 ==
  data: y output; psi input; wind_direction input; alpha_aw output; u input; v input; wind_velocity input; r input; V_aw output
function [y,alpha_aw,V_aw] = sailAngle(psi,wind_direction,u,v,wind_velocity,r)

% CoE of the sail
xs = 0;
ys = 0;
zs = 0.6;
v_t = [ wind_velocity*cos(wind_direction); wind_velocity*sin(wind_direction); 0 ];
R1 = [ cos(-psi) -sin(-psi) 0; sin(-psi) cos(-psi) 0; 0 0 1];
R2 = [ 1 0 0 ; 0 1 0; 0 0 1];
v_tb = R2*R1*v_t; % wind expressed in the body frame
V_in = [ u ; v ; 0 ];
V_awb = v_tb - V_in - cross([0;0;r],[xs;ys;zs]);
V_awu = V_awb(1);
V_awv = V_awb(2);
V_aw = V_awb(1)^2 + V_awb(2)^2;
alpha_aw = atan2(real(V_awv),real(-V_awu));

y=  0.5 * alpha_aw;

== matlab function ardupilotsailboat/MATLAB Function7 ==
  data: y output; r input; currentState input; nextState output
function [y,nextState]      = zigzag(r,currentState)
% Beta Reference Angle

switch currentState
    case 0
        if(r==1)
        nextState=1;
        else 
            nextState=0;
        end
        y=-15/180*pi;
    case 1
        if(r==1)
        nextState=0;
        else 
            nextState=1;
        end
        y=15/180*pi;
    otherwise
        y=-15/180*pi;
        nextState=0;
end

== matlab function ardupilotsailboat/MATLAB Function8 ==
  data: y output; psi input; state input
function y      = zigzagPsi(psi,state)
% Beta Reference Angle
if psi<-15 && state == 0
    y=1;
elseif psi>15 && state == 1
    y=1;
else 
    y=0;
end

== matlab function ardupilotsailboat/Subsystem1/MATLAB Function10 ==
  data: state input; y output
function y = stopSimulation(state)
if state== 6
    y=1;
else
    y=0;
end

== matlab function ardupilotsailboat/Subsystem1/MATLAB Function11 ==
  data: xw input; yw input; xs input; p_w output; ys input; xcw input; ycw input; theta output
function [p_w,theta] = passedWaypoint(xw,yw,xs,ys,xcw,ycw)
% Checking is sailboat has passed waypoint while sailing into the wind
if (ys-ycw)~= 0
theta = atan(abs(xs-xcw)/abs(ys-ycw));
else 
    theta=0;
end

p_w=0;
if xw>0 
% Angle between sail
    if (xcw-xs)<0 
        % Waypoint passed in x positive
        p_w=1;
        if(ycw-ys)<0
            % Waypoint passed in both x and y positive direction
            theta = pi + theta;
        else
            % Waypoint passed in positive x and negative y
            theta = -theta;
        end
    end 
else
    if(xcw-xs)>0 
        % Waypoint passed in x negative
        p_w=1;
        if(ycw-ys)>0
           % Waypoint passed in both x and y negative direction
        else
           % Waypoint passed in negative x and positive y
           theta= pi - theta;
        end
   end
end

== matlab function ardupilotsailboat/Subsystem1/MATLAB Function12 ==
  data: xs input; ys input; x input; y input; dist input; dist output
function dist   = travelDistance(xs,ys,x,y,dist)
% Distance Sailboat travelled

dist = dist + sqrt((xs-x)^2+(ys-y)^2);

== matlab function ardupilotsailboat/Subsystem1/MATLAB Function18 ==
  data: angle input; nextState output; currentState input
function nextState    = tack_Side(angle,currentState)
% Calculate when to tack back to waypoint

switch currentState
    case 1
        % In zone 1 can go to zone 2 and 4
        if angle < 0
            nextState=4;
        elseif angle > 15
            nextState=2;
        else 
            nextState=1;
        end
    case 2
       % In zone 2 can go to zone 3 and 1
        if angle < 15
            nextState=1;
        elseif angle > 30
            nextState=3;
        else 
            nextState=2;
        end
    case 3
        % In zone 3 can go to zone 2
        if angle < 30
            nextState=2;
        else 
            nextState=3;
        end
    case 4
       % In zone 4 can go to zone 5 and 1
        if angle > 0
            nextState=1;
        elseif angle < -15
            nextState=5;
        else 
            nextState=4;
        end
    case 5
       % In zone 5 can go to zone 6 and 4
        if angle < -30
            nextState=6;
        elseif angle >-15
            nextState=4;
        else
            nextState=5;
        end
    case 6
        % In zone 6 can go to zone 5
        if angle > -30
            nextState=5;
        else 
            nextState=6;
        end
    otherwise
        nextState=1;

end

== matlab function ardupilotsailboat/Subsystem1/MATLAB Function3 ==
  data: pathTrajectory input; y output; tack input; tackDistance output; tackLeft output; tackRight output; WA input; xtrack input; nextTackType output; indirectTackSide input; zone input; currentTackType input; currentState output; noGoAngle input; tackType input; XtrackDistance input
function [y,tackDistance, tackLeft,tackRight,nextTackType,currentState]  = headingController(pathTrajectory,tack,WA,xtrack,indirectTackSide,zone,currentTackType,noGoAngle,tackType,XtrackDistance)
% Heading State Machine

% Type of Tacks
% Direct = 1
% Indirect = 2
% Zones = 3

tackDistance = XtrackDistance;
if tack==0
    currentState = 0;
else
    % Switch between Direct and Indirect Tack and Zone Tack
    currentState = tackType;
    
end
switch currentState
    
    % Normail State 
    case 0
        y = pathTrajectory;
        nextTackType=1;
        tackLeft=0;
        tackRight=0;

    % Direct Tacking State
    case 1
       switch currentTackType
           case 1
               y=-WA*180/pi+noGoAngle;
               tackRight=1;
               tackLeft=0;
               if(xtrack>tackDistance)
                   nextTackType=0;
               else
                   nextTackType=1;
               end
               
           case 0 
               y=-WA*180/pi-noGoAngle;
               tackRight=0;
               tackLeft=1;
               if (xtrack<-tackDistance)
                   nextTackType=1;
               else 
                   nextTackType=0;
               end
           otherwise
               nextTackType=1;
               y=-WA*180/pi+45;
               tackLeft=1;
               tackRight=0;
       end
    
    % Indirect Tacking State
    case 2
        if indirectTackSide==0
             y=-WA*180/pi+noGoAngle;
        else
             y=-WA*180/pi-noGoAngle;
        end
        nextTackType=1;
        tackLeft=0;
        tackRight=0;

    % Zone Tacking State
    case 3
        switch zone
            case 1
                if currentTackType==0
                    tackLeft=1;
                    tackRight=0;
                    y=WA*180/pi-noGoAngle;
                    nextTackType=0;
                else
                    tackLeft=0;
                    tackRight=1;
                    y=WA*180/pi+noGoAngle;
                    nextTackType=1;
                end

            case 2
                if currentTackType==0
                    tackLeft=1;
                    tackRight=0;
                    y=WA*180/pi-noGoAngle;
                    nextTackType=0;
                else
                    tackLeft=0;
                    tackRight=1;
                    y=WA*180/pi+noGoAngle;
                    nextTackType=1;
                end

            case 3
                % If boat is forced in zone 3 sail past lay lines and only
                % when one has passed the lay lines sail to waypoint
                y = pathTrajectory;
                tackLeft=1;
                nextTackType=0;
                tackRight=0;
            
            case 4
                if currentTackType==0
                    tackLeft=1;
                    tackRight=0;
                    y=WA*180/pi-noGoAngle;
                    nextTackType=0;
                else
                    tackLeft=0;
                    tackRight=1;
                    y=WA*180/pi+noGoAngle;
                    nextTackType=1;
                end

            case 5
                if currentTackType==0
                    tackLeft=1;
                    tackRight=0;
                    y=WA*180/pi-noGoAngle;
                    nextTackType=0;
                else
                    tackLeft=0;
                    tackRight=1;
                    y=WA*180/pi+noGoAngle;
                    nextTackType=1;
                end

            case 6
                % Same as zone 3 just opposite tack
                y = pathTrajectory;
                tackLeft=0;
                nextTackType=1;
                tackRight=1;

            otherwise
                y = pathTrajectory;
                nextTackType=0;
                tackLeft=1;
                tackRight=0;
        end

    otherwise
        y=0;
        nextTackType=2;
        tackLeft=0;
        tackRight=0;

end
if currentState==3
    if tackLeft==1
         y=WA*180/pi-noGoAngle;
         nextTackType=0;
    else
         y=WA*180/pi+noGoAngle;
         nextTackType=1;
    end
end

== matlab function ardupilotsailboat/Subsystem1/MATLAB Function4 ==
  data: R input; nextState output; currentWaypoint output; currentState input
function [nextState,currentWaypoint]  = wayPointController(R,currentState)
% Waypoint switching
% With each added waypoint another case should be added
switch currentState
    % First waypoint
    case 0
        % Check if waypoint lies within radius of acceptance
        if(R==1)
            % Switch current Waypoint to next waypoint
            nextState=1;
            currentWaypoint=1;
        % Waypoint not reached
        else
            nextState=0;
            currentWaypoint=0;
        end
    case 1
        % Check if waypoint lies within radius of acceptance
        if(R==1)
            % Switch current Waypoint to next waypoint
            nextState=2;
            currentWaypoint=2;
       % Waypoint not reached
       else
            nextState=currentState;
            currentWaypoint=1;
       end
    case 2
       % Check if waypoint lies within radius of acceptance
       if(R==1)
            % Switch current Waypoint to next waypoint
            nextState=3;
            currentWaypoint=3;
       % Waypoint not reached
       else
            nextState=currentState;
            currentWaypoint=2;
       end
     case 3
       % Check if waypoint lies within radius of acceptance
       if(R==1)
            % Switch current Waypoint to next waypoint
            nextState=4;
            currentWaypoint=4;
       % Waypoint not reached 
       else
            nextState=currentState;
            currentWaypoint=3;
       end
     case 4
       % Check if waypoint lies within radius of acceptance
       if(R==1)
            % Switch current Waypoint to next waypoint
            nextState=5;
            currentWaypoint=5;
       % Waypoint not reached
       else
            nextState=currentState;
            currentWaypoint=4;
       end
       case 5
       % Check if waypoint lies within radius of acceptance
       if(R==1)
            % Switch current Waypoint to next waypoint
            nextState=0;
            currentWaypoint=0;
       % Waypoint not reached
       else
            nextState=currentState;
            currentWaypoint=5;
       end
    otherwise
        nextState=0;
        currentWaypoint=0;
end

== matlab function ardupilotsailboat/Subsystem1/MATLAB Function5 ==
  data: xWaypoint input; yWaypoint input; xBoat input; yBoat input; R input; acceptance output
function acceptance   = circleOfAcceptanceController(xWaypoint,yWaypoint,xBoat,yBoat,R)
    if (sqrt((abs(xWaypoint-xBoat))^2+(abs(yWaypoint-yBoat))^2)<R)
        acceptance=1;
    else
        acceptance=0;
    end
end

== matlab function ardupilotsailboat/Subsystem1/MATLAB Function6 ==
  data: xw input; yw input; xwp input; y output; ywp input
function y  = distanceToWaypoint(xw,yw,xwp,ywp)
% Calculate distance to waypoint
y = (sqrt((ywp-yw)^2+(xwp-xw)^2))/2;

== matlab function ardupilotsailboat/Subsystem1/MATLAB Function7 ==
  data: wa input; y output; psi input; w output; p output; awa output
function [y,w,p,awa]   = apparentWindAngle(wa,psi)
% Calculate Apparent Wind Angle
if psi> pi
    psi= psi-2*pi;
else
    if psi<-pi
    psi=psi+2*pi;
    end
end
awa = psi+wa;
p=psi;
w= wa;

if abs(awa)<pi/4
    y=1;
else

    y=0;
end

== matlab function ardupilotsailboat/Subsystem1/MATLAB Function8 ==
  data: x1 input; y1 input; u input; y output; us input
function y = controlAngle(x1,y1,u,us)
ys=0;
if x1>=0 && y1>=0
    ys=u;
elseif x1>=0 && y1<=0
        ys=pi-u;
elseif x1==0 && y1>0
        ys=0;
elseif x1==0 && y1<0
        ys=pi;
elseif y1==0 && x1>0
        ys=pi/2;
elseif y1==0 && x1<0
        ys=-pi/2;
elseif x1<0 && y1>0
    ys=-u;
elseif x1<0 && y1<0
    ys=-pi+u;
else
    ys=u;
end
if (ys-us)<-pi
    y = ys+2*pi;
elseif (ys-us)>pi
    y=ys-2*pi;
else
    y=ys;
end

== matlab function ardupilotsailboat/Subsystem1/MATLAB Function9 ==
  data: angle output; dist input; xtrack input; currentState input; tack output; nextState output; windDirection input; wayPointHeading input
function [angle,tack,nextState]  = tackAngle(dist,xtrack,currentState,windDirection,wayPointHeading)
% Calculate when to tack back to waypoint
if dist ~= 0
    angle = atan(xtrack/dist);
else
    angle=0;
end

if windDirection > pi
    windDirection = windDirection - pi;
else
    if windDirection < -pi
        windDirection = windDirection + pi;
    end
end

if wayPointHeading > pi
    wayPointHeading = wayPointHeading - pi;
else
    if wayPointHeading < -pi
        wayPointHeading = wayPointHeading + pi;
    end
end

angle = angle * (180/pi) - (windDirection-wayPointHeading);

% tack == 0 is left tack
% tack == 1 is right tack
switch currentState
    case 0
        tack=0;
        if angle>=45
            nextState=1;
        else
            nextState=0;
        end
    case 1
        tack=1;
        if angle<=-45
            nextState=0;
        else
            nextState=1;
        end

    otherwise
        tack=0;
        nextState=0;

end
